simulink model "GFLIB_Hyst_BAM_F32"  (Simulink 7.3)
settings: Solver=ode45  StartTime=0.0  StopTime=10.0  RelTol=1e-3
undefined symbols (not defined in the file): f32HystOff, f32HystOn, f32OutValOff, f32OutValOn
settings Model: Creator=B17364  LastModifiedBy=B17364

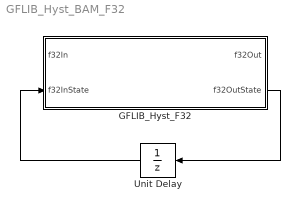
== system GFLIB_Hyst_BAM_F32 ==
  GFLIB_Hyst_F32 : Subsystem  mask(GFLIB_Hyst_F32){f32HystOn=f32HystOn, f32HystOff=f32HystOff, f32OutValOn=f32OutValOn, f32OutValOff=f32OutValOff}
      mask help: Bit accurate model of hysteresis function. All parameters as well as input and output are 32-bit integers.
      mask init:
      | pos = get_param(gcb, 'Position');width = pos(3) - pos(1); height = pos(4) - pos(2);tX=width/2;tY=height*0.9;
      mask Display: color('black');port_label('input',1,'f32In');port_label('input',2,'f32InState');port_label('output',1,'f32Out');port_label('output',2,'f32OutState');color('black');disp('GFLIB_Hyst_F32');color('blue');text(tX,tY, 'BAM', 'horizontalAlignment', 'center');
  Unit Delay : UnitDelay  SampleTime=-1
  wires:
  GFLIB_Hyst_F32/2(f32OutState) -> Unit Delay/1
  Unit Delay/1 -> GFLIB_Hyst_F32/2(f32InState)

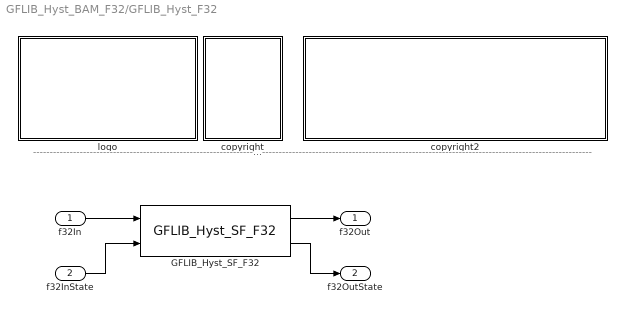
== system GFLIB_Hyst_BAM_F32/GFLIB_Hyst_F32 ==
  note: ---------------------------------------------------------------------------------------------------------------------------------------------------------------------------------------------------
  f32In : Inport  OutDataType=fixdt(1, 16)  OutScaling=2^0
  f32InState : Inport  Port=2  OutDataType=fixdt(1, 16)  OutScaling=2^0
  GFLIB_Hyst_SF_F32 : S-Function  FunctionName=GFLIB_Hyst_SF_F32  Parameters=f32HystOn,f32HystOff,f32OutValOn,f32OutValOff  EnableBusSupport=off
  copyright : Subsystem
      mask Display: text(10,90,'FILE:');text(10,75,'DESRIPTION:')text(10,60,'COPYRIGHT:')text(10,45,'VERSION:')text(10,30,'DATE:')
  copyright2 : Subsystem
      mask Display: text(10,90,'GFLIB_Hyst_BAM_F32.mdl');text(10,75,'Hysteresis function.');text(10,60,'Freescale')text(10,45,'0.1');text(10,30,'09-Apr-2014');
  logo : Subsystem
      mask Display: image(imread('logo.jpg'))
  f32Out : Outport  OutDataType=fixdt(1, 16)  OutScaling=2^0
  f32OutState : Outport  Port=2  OutDataType=fixdt(1, 16)  OutScaling=2^0
  wires:
  f32In/1 -> GFLIB_Hyst_SF_F32/1
  GFLIB_Hyst_SF_F32/1 -> f32Out/1
  f32InState/1 -> GFLIB_Hyst_SF_F32/2
  GFLIB_Hyst_SF_F32/2 -> f32OutState/1

== system GFLIB_Hyst_BAM_F32/GFLIB_Hyst_F32/copyright ==

== system GFLIB_Hyst_BAM_F32/GFLIB_Hyst_F32/copyright2 ==

== system GFLIB_Hyst_BAM_F32/GFLIB_Hyst_F32/logo ==
